simulink model "convertTemperture_CtoF_"  (R2021a)
settings: Solver=VariableStepAuto  StartTime=0.0  StopTime=50  MaxStep=1e-6  RelTol=1e-3
settings Model: Creator=HP  LastModifiedBy=HP

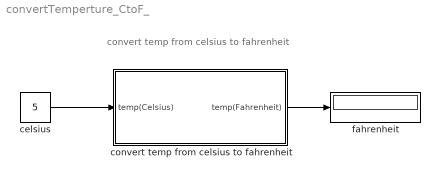
== system convertTemperture_CtoF_ ==
  note: convert temp from celsius to fahrenheit
  celsius : Constant  Value=5
  convert temp from celsius to fahrenheit : Subsystem
  fahrenheit : Display
  wires:
  celsius/1 -> convert temp from celsius to fahrenheit/1(temp(Celsius))
  convert temp from celsius to fahrenheit/1(temp(Fahrenheit)) -> fahrenheit/1

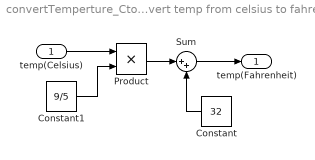
== system convertTemperture_CtoF_/convert temp from celsius to fahrenheit ==
  temp(Celsius) : Inport
  Constant : Constant  Value=32
  Constant1 : Constant  Value=9/5
  Product : Product
  Sum : Sum  Inputs=|++
  temp(Fahrenheit) : Outport
  wires:
  temp(Celsius)/1 -> Product/1
  Constant1/1 -> Product/2
  Constant/1 -> Sum/2
  Product/1 -> Sum/1
  Sum/1 -> temp(Fahrenheit)/1
